simulink model "octave1"  (R2015a)
settings: Solver=ode45  StartTime=0.0  StopTime=10.0  RelTol=1e-3
InitFcn:
  | %% DSPBuilder Start
  | alt_dspbuilder_update_model(bdroot)
  | %% DSPBuilder End
libraries: allblocks_alteradspbuilder2 x1175
(part 2 of 16)

== system octave1/GradOrien/sub_GradOrian ==
  L_y_add_1 : Inport
  L_x_add_1 : Inport  Port=2
  L_x_sub_1 : Inport  Port=3
  L_y_sub_1 : Inport  Port=4
  AltBus : allblocks_alteradspbuilder2/AltBus  BusType=Unsigned Integer  bwl=9  bwr=0  saturate=off  floatingPointInput=on  floatingPointOutput=on  logOutputs=off  logFile=C:\Users\ASUS\Desktop\sift_fpga_final\Octave_1\tb_octave1\octave1_GradOrien_sub%5FGradOrian_AltBus.fixedpointlog
  Bus Builder : allblocks_alteradspbuilder2/Bus Builder  BusType=Unsigned Integer  bwl=3  bwr=1  pipeline_display=0
  Comparator3 : allblocks_alteradspbuilder2/Comparator  direction=a > b  pipeline_display=0  allowFloatingPointOverride=on  logOutputs=off  logFile=C:\Users\ASUS\Desktop\sift_fpga_final\Octave_1\tb_octave1\octave1_GradOrien_sub%5FGradOrian_Comparator3.fixedpointlog
  Comparator4 : allblocks_alteradspbuilder2/Comparator  direction=a > b  pipeline_display=0  allowFloatingPointOverride=on  logOutputs=off  logFile=C:\Users\ASUS\Desktop\sift_fpga_final\Octave_1\tb_octave1\octave1_GradOrien_sub%5FGradOrian_Comparator4.fixedpointlog
  Comparator5 : allblocks_alteradspbuilder2/Comparator  direction=a > b  pipeline_display=0  allowFloatingPointOverride=on  logOutputs=off  logFile=C:\Users\ASUS\Desktop\sift_fpga_final\Octave_1\tb_octave1\octave1_GradOrien_sub%5FGradOrian_Comparator5.fixedpointlog
  Constant : allblocks_alteradspbuilder2/Constant  mask_cst=5  BusType=Unsigned Integer  bwl=8  bwr=0  roundMode=Truncate  satMode=Wrap  SpecifyClock=off  allowFloatingPointOverride=on  logOutputs=off  logFile=C:\Users\ASUS\Desktop\sift_fpga_final\Octave_1\tb_octave1\octave1_GradOrien_sub%5FGradOrian_Constant.fixedpointlog
  Constant1 : allblocks_alteradspbuilder2/Constant  mask_cst=4  BusType=Unsigned Integer  bwl=8  bwr=0  roundMode=Truncate  satMode=Wrap  SpecifyClock=off  allowFloatingPointOverride=on  logOutputs=off  logFile=C:\Users\ASUS\Desktop\sift_fpga_final\Octave_1\tb_octave1\octave1_GradOrien_sub%5FGradOrian_Constant1.fixedpointlog
  Constant2 : allblocks_alteradspbuilder2/Constant  mask_cst=7  BusType=Unsigned Integer  bwl=8  bwr=0  roundMode=Truncate  satMode=Wrap  SpecifyClock=off  allowFloatingPointOverride=on  logOutputs=off  logFile=C:\Users\ASUS\Desktop\sift_fpga_final\Octave_1\tb_octave1\octave1_GradOrien_sub%5FGradOrian_Constant2.fixedpointlog
  Constant3 : allblocks_alteradspbuilder2/Constant  mask_cst=1  BusType=Unsigned Integer  bwl=8  bwr=0  roundMode=Truncate  satMode=Wrap  SpecifyClock=off  allowFloatingPointOverride=on  logOutputs=off  logFile=C:\Users\ASUS\Desktop\sift_fpga_final\Octave_1\tb_octave1\octave1_GradOrien_sub%5FGradOrian_Constant3.fixedpointlog
  Constant4 : allblocks_alteradspbuilder2/Constant  mask_cst=6  BusType=Unsigned Integer  bwl=8  bwr=0  roundMode=Truncate  satMode=Wrap  SpecifyClock=off  allowFloatingPointOverride=on  logOutputs=off  logFile=C:\Users\ASUS\Desktop\sift_fpga_final\Octave_1\tb_octave1\octave1_GradOrien_sub%5FGradOrian_Constant4.fixedpointlog
  Constant5 : allblocks_alteradspbuilder2/Constant  mask_cst=3  BusType=Unsigned Integer  bwl=8  bwr=0  roundMode=Truncate  satMode=Wrap  SpecifyClock=off  allowFloatingPointOverride=on  logOutputs=off  logFile=C:\Users\ASUS\Desktop\sift_fpga_final\Octave_1\tb_octave1\octave1_GradOrien_sub%5FGradOrian_Constant5.fixedpointlog
  Constant6 : allblocks_alteradspbuilder2/Constant  mask_cst=8  BusType=Unsigned Integer  bwl=8  bwr=0  roundMode=Truncate  satMode=Wrap  SpecifyClock=off  allowFloatingPointOverride=on  logOutputs=off  logFile=C:\Users\ASUS\Desktop\sift_fpga_final\Octave_1\tb_octave1\octave1_GradOrien_sub%5FGradOrian_Constant6.fixedpointlog
  Constant7 : allblocks_alteradspbuilder2/Constant  mask_cst=2  BusType=Unsigned Integer  bwl=8  bwr=0  roundMode=Truncate  satMode=Wrap  SpecifyClock=off  allowFloatingPointOverride=on  logOutputs=off  logFile=C:\Users\ASUS\Desktop\sift_fpga_final\Octave_1\tb_octave1\octave1_GradOrien_sub%5FGradOrian_Constant7.fixedpointlog
  Delay : allblocks_alteradspbuilder2/Delay  pipeline=1  pipeline_display=1  ClockPhase=1  use_ena=on  use_sclr=off  allowFloatingPointOverride=on  logOutputs=off  logFile=C:\Users\ASUS\Desktop\sift_fpga_final\Octave_1\tb_octave1\octave1_GradOrien_sub%5FGradOrian_Delay.fixedpointlog  use_init=off  reset_value=1
  Delay1 : allblocks_alteradspbuilder2/Delay  pipeline=1  pipeline_display=1  ClockPhase=1  use_ena=on  use_sclr=off  allowFloatingPointOverride=on  logOutputs=off  logFile=C:\Users\ASUS\Desktop\sift_fpga_final\Octave_1\tb_octave1\octave1_GradOrien_sub%5FGradOrian_Delay1.fixedpointlog  use_init=off  reset_value=1
  Delay2 : allblocks_alteradspbuilder2/Delay  pipeline=1  pipeline_display=1  ClockPhase=1  use_ena=on  use_sclr=off  allowFloatingPointOverride=on  logOutputs=off  logFile=C:\Users\ASUS\Desktop\sift_fpga_final\Octave_1\tb_octave1\octave1_GradOrien_sub%5FGradOrian_Delay2.fixedpointlog  use_init=off  reset_value=1
  Multiplexer2 : allblocks_alteradspbuilder2/Multiplexer  numInputs=8  pipeline=0  oneHot=off  pipeline_display=0  use_ena=off  use_aclr=off  allowFloatingPointOverride=on  logOutputs=off  logFile=C:\Users\ASUS\Desktop\sift_fpga_final\Octave_1\tb_octave1\octave1_GradOrien_sub%5FGradOrian_Multiplexer2.fixedpointlog
  Multiplexer3 : allblocks_alteradspbuilder2/Multiplexer  numInputs=2  pipeline=0  oneHot=off  pipeline_display=0  use_ena=off  use_aclr=off  allowFloatingPointOverride=on  logOutputs=off  logFile=C:\Users\ASUS\Desktop\sift_fpga_final\Octave_1\tb_octave1\octave1_GradOrien_sub%5FGradOrian_Multiplexer3.fixedpointlog
  Multiplexer4 : allblocks_alteradspbuilder2/Multiplexer  numInputs=2  pipeline=0  oneHot=off  pipeline_display=0  use_ena=off  use_aclr=off  allowFloatingPointOverride=on  logOutputs=off  logFile=C:\Users\ASUS\Desktop\sift_fpga_final\Octave_1\tb_octave1\octave1_GradOrien_sub%5FGradOrian_Multiplexer4.fixedpointlog
  Parallel Adder Subtractor : allblocks_alteradspbuilder2/Parallel Adder Subtractor  number_of_inputs=2  direction=+-  use_pipeline=on  pipeline_display=1  phase_selection=1  use_ena=on  use_aclr=off  allowFloatingPointOverride=on  logOutputs=off  logFile=C:\Users\ASUS\Desktop\sift_fpga_final\Octave_1\tb_octave1\octave1_GradOrien_sub%5FGradOrian_Parallel+Adder+Subtractor.fixedpointlog
  Parallel Adder Subtractor1 : allblocks_alteradspbuilder2/Parallel Adder Subtractor  number_of_inputs=2  direction=+-  use_pipeline=on  pipeline_display=1  phase_selection=1  use_ena=on  use_aclr=off  allowFloatingPointOverride=on  logOutputs=off  logFile=C:\Users\ASUS\Desktop\sift_fpga_final\Octave_1\tb_octave1\octave1_GradOrien_sub%5FGradOrian_Parallel+Adder+Subtractor1.fixedpointlog
  Parallel Adder Subtractor2 : allblocks_alteradspbuilder2/Parallel Adder Subtractor  number_of_inputs=2  direction=-+  use_pipeline=on  pipeline_display=1  phase_selection=1  use_ena=on  use_aclr=off  allowFloatingPointOverride=on  logOutputs=off  logFile=C:\Users\ASUS\Desktop\sift_fpga_final\Octave_1\tb_octave1\octave1_GradOrien_sub%5FGradOrian_Parallel+Adder+Subtractor2.fixedpointlog
  Parallel Adder Subtractor3 : allblocks_alteradspbuilder2/Parallel Adder Subtractor  number_of_inputs=2  direction=-+  use_pipeline=on  pipeline_display=1  phase_selection=1  use_ena=on  use_aclr=off  allowFloatingPointOverride=on  logOutputs=off  logFile=C:\Users\ASUS\Desktop\sift_fpga_final\Octave_1\tb_octave1\octave1_GradOrien_sub%5FGradOrian_Parallel+Adder+Subtractor3.fixedpointlog
  Parallel Adder Subtractor5 : allblocks_alteradspbuilder2/Parallel Adder Subtractor  number_of_inputs=2  direction=++  use_pipeline=on  pipeline_display=1  phase_selection=1  use_ena=on  use_aclr=off  allowFloatingPointOverride=on  logOutputs=off  logFile=C:\Users\ASUS\Desktop\sift_fpga_final\Octave_1\tb_octave1\octave1_GradOrien_sub%5FGradOrian_Parallel+Adder+Subtractor5.fixedpointlog
  orien : Outport
  m_xy : Outport  Port=2
  wires:
  Multiplexer2/1 -> Delay2/1
  Bus Builder/1 -> Multiplexer2/1
  Delay2/1 -> orien/1
  Constant6/1 -> Multiplexer2/8
  Constant4/1 -> Multiplexer2/6
  Constant5/1 -> Multiplexer2/7
  Comparator3/1 -> Delay/1
  Constant7/1 -> Multiplexer2/9
  [L_y_sub_1] -> Comparator4/2
  [L_x_sub_1] -> Comparator3/2
  [L_y_add_1] -> Comparator4/1
  [L_x_add_1] -> Comparator3/1
  [Ly_1] -> Multiplexer4/2
  Delay1/1 -> Bus Builder/2, Multiplexer4/1
  [Lx] -> Multiplexer3/3
  Delay/1 -> Bus Builder/1, Multiplexer3/1
  [Lx_1] -> Multiplexer3/2
  [Ly] -> Multiplexer4/3
  Constant/1 -> Multiplexer2/2
  [clken] -> Delay1/2
  Comparator5/1 -> Bus Builder/3
  [clken] -> Delay/2
  Comparator4/1 -> Delay1/1
  Multiplexer4/1 -> Comparator5/2, Parallel Adder Subtractor5/2
  Multiplexer3/1 -> Comparator5/1, Parallel Adder Subtractor5/1
  [clken] -> Parallel Adder Subtractor5/3
  Parallel Adder Subtractor5/1 -> AltBus/1
  [clken] -> Delay2/2
  Constant1/1 -> Multiplexer2/3
  Parallel Adder Subtractor2/1 -> [Lx_1]
  [clken] -> Parallel Adder Subtractor2/3
  [L_y_add_1] -> Parallel Adder Subtractor3/1
  Parallel Adder Subtractor3/1 -> [Ly_1]
  [L_y_sub_1] -> Parallel Adder Subtractor3/2
  [L_x_sub_1] -> Parallel Adder Subtractor2/2
  [clken] -> Parallel Adder Subtractor3/3
  [L_x_add_1] -> Parallel Adder Subtractor2/1
  [L_x_sub_1] -> Parallel Adder Subtractor/2
  [L_y_sub_1] -> Parallel Adder Subtractor1/2
  [L_y_add_1] -> Parallel Adder Subtractor1/1
  [clken] -> Parallel Adder Subtractor/3
  Parallel Adder Subtractor/1 -> [Lx]
  Parallel Adder Subtractor1/1 -> [Ly]
  [clken] -> Parallel Adder Subtractor1/3
  [L_x_add_1] -> Parallel Adder Subtractor/1
  Constant2/1 -> Multiplexer2/4
  Constant3/1 -> Multiplexer2/5
  L_x_add_1/1 -> [L_x_add_1]
  L_x_sub_1/1 -> [L_x_sub_1]
  L_y_add_1/1 -> [L_y_add_1]
  L_y_sub_1/1 -> [L_y_sub_1]
  AltBus/1 -> m_xy/1

== system octave1/calculate_key_point/find_KeyPoint ==
  dataIn_10 : Inport
  dataIn_11 : Inport  Port=2
  dataIn_12 : Inport  Port=3
  dataIn_13 : Inport  Port=4
  dataIn_14 : Inport  Port=5
  dataIn_15 : Inport  Port=6
  dataIn_16 : Inport  Port=7
  dataIn_17 : Inport  Port=8
  dataIn_18 : Inport  Port=9
  dataIn_20 : Inport  Port=10
  dataIn_21 : Inport  Port=11
  dataIn_22 : Inport  Port=12
  dataIn_23 : Inport  Port=13
  dataIn_24 : Inport  Port=14
  dataIn_25 : Inport  Port=15
  dataIn_26 : Inport  Port=16
  dataIn_27 : Inport  Port=17
  dataIn_28 : Inport  Port=18
  dataIn_30 : Inport  Port=19
  dataIn_31 : Inport  Port=20
  dataIn_32 : Inport  Port=21
  dataIn_33 : Inport  Port=22
  dataIn_34 : Inport  Port=23
  dataIn_35 : Inport  Port=24
  dataIn_36 : Inport  Port=25
  dataIn_37 : Inport  Port=26
  dataIn_38 : Inport  Port=27
  Logical Bit Operator : allblocks_alteradspbuilder2/Logical Bit Operator  LogicalOperator=OR  user_inputs=2  pipeline_display=0
  find_Keymax : Subsystem
  find_min : Subsystem
  is_KeyPoint : Outport
  wires:
  [dataIn_32] -> find_Keymax/21(dataIn_32)
  [dataIn_33] -> find_Keymax/22(dataIn_33)
  [dataIn_36] -> find_Keymax/25(dataIn_36)
  [dataIn_37] -> find_Keymax/26(dataIn_37)
  [dataIn_34] -> find_Keymax/23(dataIn_34)
  [dataIn_35] -> find_Keymax/24(dataIn_35)
  [dataIn_30] -> find_Keymax/19(dataIn_30)
  [dataIn_31] -> find_Keymax/20(dataIn_31)
  [is_KeyPoint_Max] -> Logical Bit Operator/2
  [is_KeyPoint_Min] -> Logical Bit Operator/1
  find_Keymax/1(is_KeyPoint) -> [is_KeyPoint_Max]
  [dataIn_28] -> find_Keymax/18(dataIn_28)
  [dataIn_26] -> find_Keymax/16(dataIn_26)
  [dataIn_22] -> find_Keymax/12(dataIn_22)
  [dataIn_27] -> find_Keymax/17(dataIn_27)
  [dataIn_20] -> find_Keymax/10(dataIn_20)
  [dataIn_23] -> find_Keymax/13(dataIn_23)
  [dataIn_24] -> find_Keymax/14(dataIn_24)
  [dataIn_21] -> find_Keymax/11(dataIn_21)
  [dataIn_25] -> find_Keymax/15(dataIn_25)
  [dataIn_10] -> find_Keymax/1(dataIn_10)
  [dataIn_11] -> find_Keymax/2(dataIn_11)
  [dataIn_12] -> find_Keymax/3(dataIn_12)
  dataIn_23/1 -> [dataIn_23]
  dataIn_17/1 -> [dataIn_17]
  dataIn_22/1 -> [dataIn_22]
  dataIn_14/1 -> [dataIn_14]
  dataIn_16/1 -> [dataIn_16]
  dataIn_28/1 -> [dataIn_28]
  dataIn_20/1 -> [dataIn_20]
  dataIn_21/1 -> [dataIn_21]
  dataIn_26/1 -> [dataIn_26]
  dataIn_10/1 -> [dataIn_10]
  dataIn_30/1 -> [dataIn_30]
  dataIn_27/1 -> [dataIn_27]
  dataIn_25/1 -> [dataIn_25]
  dataIn_15/1 -> [dataIn_15]
  dataIn_18/1 -> [dataIn_18]
  dataIn_24/1 -> [dataIn_24]
  dataIn_32/1 -> [dataIn_32]
  dataIn_13/1 -> [dataIn_13]
  dataIn_31/1 -> [dataIn_31]
  [dataIn_14] -> find_Keymax/5(dataIn_14)
  dataIn_34/1 -> [dataIn_34]
  dataIn_11/1 -> [dataIn_11]
  [dataIn_17] -> find_Keymax/8(dataIn_17)
  dataIn_35/1 -> [dataIn_35]
  dataIn_33/1 -> [dataIn_33]
  dataIn_38/1 -> [dataIn_38]
  [dataIn_13] -> find_Keymax/4(dataIn_13)
  [dataIn_16] -> find_Keymax/7(dataIn_16)
  [dataIn_15] -> find_Keymax/6(dataIn_15)
  dataIn_12/1 -> [dataIn_12]
  [dataIn_18] -> find_Keymax/9(dataIn_18)
  dataIn_36/1 -> [dataIn_36]
  dataIn_37/1 -> [dataIn_37]
  [dataIn_38] -> find_Keymax/27(dataIn_38)
  find_min/1(is_KeyPoint) -> [is_KeyPoint_Min]
  [dataIn_11] -> find_min/2(dataIn_11)
  [dataIn_12] -> find_min/3(dataIn_12)
  [dataIn_13] -> find_min/4(dataIn_13)
  [dataIn_15] -> find_min/6(dataIn_15)
  [dataIn_16] -> find_min/7(dataIn_16)
  [dataIn_17] -> find_min/8(dataIn_17)
  [dataIn_18] -> find_min/9(dataIn_18)
  [dataIn_31] -> find_min/20(dataIn_31)
  [dataIn_14] -> find_min/5(dataIn_14)
  [is_KeyPoint] -> is_KeyPoint/1
  [dataIn_33] -> find_min/22(dataIn_33)
  [dataIn_32] -> find_min/21(dataIn_32)
  [dataIn_34] -> find_min/23(dataIn_34)
  [dataIn_35] -> find_min/24(dataIn_35)
  [dataIn_36] -> find_min/25(dataIn_36)
  [dataIn_21] -> find_min/11(dataIn_21)
  [dataIn_22] -> find_min/12(dataIn_22)
  [dataIn_23] -> find_min/13(dataIn_23)
  [dataIn_25] -> find_min/15(dataIn_25)
  [dataIn_24] -> find_min/14(dataIn_24)
  [dataIn_38] -> find_min/27(dataIn_38)
  [dataIn_20] -> find_min/10(dataIn_20)
  [dataIn_26] -> find_min/16(dataIn_26)
  [dataIn_30] -> find_min/19(dataIn_30)
  [dataIn_27] -> find_min/17(dataIn_27)
  [dataIn_37] -> find_min/26(dataIn_37)
  [dataIn_28] -> find_min/18(dataIn_28)
  [dataIn_10] -> find_min/1(dataIn_10)
  Logical Bit Operator/1 -> [is_KeyPoint]

== system octave1/calculate_key_point/line_buff_3x3 ==
  dataIn : Inport
  clken : Inport  Port=2
  Delay : allblocks_alteradspbuilder2/Delay  pipeline=1  pipeline_display=1  ClockPhase=1  use_ena=on  use_sclr=off  allowFloatingPointOverride=on  logOutputs=off  logFile=C:\Users\ASUS\Desktop\sift_fpga_final\Octave_1\find_key_point\tb_calculate_key_points\calculate%5Fkey%5Fpoints_calculate%5Fkey%5Fpoint_line%5Fbuff%5F3x3_Delay.fixedpointlog  use_init=off  reset_value=1
  Delay1 : allblocks_alteradspbuilder2/Delay  pipeline=1  pipeline_display=1  ClockPhase=1  use_ena=on  use_sclr=off  allowFloatingPointOverride=on  logOutputs=off  logFile=C:\Users\ASUS\Desktop\sift_fpga_final\Octave_1\find_key_point\tb_calculate_key_points\calculate%5Fkey%5Fpoints_calculate%5Fkey%5Fpoint_line%5Fbuff%5F3x3_Delay1.fixedpointlog  use_init=off  reset_value=1
  Delay10 : allblocks_alteradspbuilder2/Delay  pipeline=1  pipeline_display=1  ClockPhase=1  use_ena=on  use_sclr=off  allowFloatingPointOverride=on  logOutputs=off  logFile=C:\Users\ASUS\Desktop\sift_fpga_final\Octave_1\find_key_point\tb_calculate_key_points\calculate%5Fkey%5Fpoints_calculate%5Fkey%5Fpoint_line%5Fbuff%5F3x3_Delay10.fixedpointlog  use_init=off  reset_value=1
  Delay2 : allblocks_alteradspbuilder2/Delay  pipeline=1  pipeline_display=1  ClockPhase=1  use_ena=on  use_sclr=off  allowFloatingPointOverride=on  logOutputs=off  logFile=C:\Users\ASUS\Desktop\sift_fpga_final\Octave_1\find_key_point\tb_calculate_key_points\calculate%5Fkey%5Fpoints_calculate%5Fkey%5Fpoint_line%5Fbuff%5F3x3_Delay2.fixedpointlog  use_init=off  reset_value=1
  Delay5 : allblocks_alteradspbuilder2/Delay  pipeline=1  pipeline_display=1  ClockPhase=1  use_ena=on  use_sclr=off  allowFloatingPointOverride=on  logOutputs=off  logFile=C:\Users\ASUS\Desktop\sift_fpga_final\Octave_1\find_key_point\tb_calculate_key_points\calculate%5Fkey%5Fpoints_calculate%5Fkey%5Fpoint_line%5Fbuff%5F3x3_Delay5.fixedpointlog  use_init=off  reset_value=1
  Delay6 : allblocks_alteradspbuilder2/Delay  pipeline=1  pipeline_display=1  ClockPhase=1  use_ena=on  use_sclr=off  allowFloatingPointOverride=on  logOutputs=off  logFile=C:\Users\ASUS\Desktop\sift_fpga_final\Octave_1\find_key_point\tb_calculate_key_points\calculate%5Fkey%5Fpoints_calculate%5Fkey%5Fpoint_line%5Fbuff%5F3x3_Delay6.fixedpointlog  use_init=off  reset_value=1
  Delay9 : allblocks_alteradspbuilder2/Delay  pipeline=1  pipeline_display=1  ClockPhase=1  use_ena=on  use_sclr=off  allowFloatingPointOverride=on  logOutputs=off  logFile=C:\Users\ASUS\Desktop\sift_fpga_final\Octave_1\find_key_point\tb_calculate_key_points\calculate%5Fkey%5Fpoints_calculate%5Fkey%5Fpoint_line%5Fbuff%5F3x3_Delay9.fixedpointlog  use_init=off  reset_value=1
  Memory Delay : allblocks_alteradspbuilder2/Memory Delay  BusType=Unsigned Integer  bwl=8  bwr=0  pipeline=638  pipeline_display=638  ram_type=AUTO  use_ena=on  use_sclr=off  allowFloatingPointOverride=on  logOutputs=off  logFile=C:\Users\ASUS\Desktop\sift_fpga_final\Octave_1\find_key_point\tb_calculate_key_points\calculate%5Fkey%5Fpoints_calculate%5Fkey%5Fpoint_line%5Fbuff%5F3x3_Memory+Delay.fixedpointlog
  Memory Delay1 : allblocks_alteradspbuilder2/Memory Delay  BusType=Unsigned Integer  bwl=8  bwr=0  pipeline=638  pipeline_display=638  ram_type=AUTO  use_ena=on  use_sclr=off  allowFloatingPointOverride=on  logOutputs=off  logFile=C:\Users\ASUS\Desktop\sift_fpga_final\Octave_1\find_key_point\tb_calculate_key_points\calculate%5Fkey%5Fpoints_calculate%5Fkey%5Fpoint_line%5Fbuff%5F3x3_Memory+Delay1.fixedpointlog
  Out00 : Outport
  Out01 : Outport  Port=2
  Out02 : Outport  Port=3
  Out10 : Outport  Port=4
  Out11 : Outport  Port=5
  Out12 : Outport  Port=6
  Out20 : Outport  Port=7
  Out21 : Outport  Port=8
  Out22 : Outport  Port=9
  wires:
  Delay1/1 -> [data_01], Delay2/1
  Delay/1 -> [data_00], Delay1/1
  Delay9/1 -> [data_21], Delay10/1
  [clken] -> Delay10/2
  [clken] -> Memory Delay1/2
  Delay6/1 -> Memory Delay1/1, [data_12]
  Memory Delay1/1 -> [data_20], Delay9/1
  [clken] -> Delay9/2
  [data_02] -> Out02/1
  [clken] -> Delay1/2
  [clken] -> Delay/2
  [data_in] -> Delay/1
  [clken] -> Delay2/2
  Delay2/1 -> Memory Delay/1, [data_02]
  [data_22] -> Out22/1
  Delay10/1 -> [data_22]
  clken/1 -> [clken]
  [data_21] -> Out21/1
  [data_20] -> Out20/1
  [data_10] -> Out10/1
  Memory Delay/1 -> [data_10], Delay5/1
  [clken] -> Memory Delay/2
  [clken] -> Delay6/2
  Delay5/1 -> [data_11], Delay6/1
  [data_12] -> Out12/1
  [data_00] -> Out00/1
  [data_01] -> Out01/1
  [clken] -> Delay5/2
  [data_11] -> Out11/1
  dataIn/1 -> [data_in]

== system octave1/calculate_key_point/line_buff_3x3(1) ==
  dataIn : Inport
  clken : Inport  Port=2
  Delay : allblocks_alteradspbuilder2/Delay  pipeline=1  pipeline_display=1  ClockPhase=1  use_ena=on  use_sclr=off  allowFloatingPointOverride=on  logOutputs=off  logFile=C:\Users\ASUS\Desktop\sift_fpga_final\Octave_1\find_key_point\tb_calculate_key_points\calculate%5Fkey%5Fpoints_calculate%5Fkey%5Fpoint_line%5Fbuff%5F3x3%281%29_Delay.fixedpointlog  use_init=off  reset_value=1
  Delay1 : allblocks_alteradspbuilder2/Delay  pipeline=1  pipeline_display=1  ClockPhase=1  use_ena=on  use_sclr=off  allowFloatingPointOverride=on  logOutputs=off  logFile=C:\Users\ASUS\Desktop\sift_fpga_final\Octave_1\find_key_point\tb_calculate_key_points\calculate%5Fkey%5Fpoints_calculate%5Fkey%5Fpoint_line%5Fbuff%5F3x3%281%29_Delay1.fixedpointlog  use_init=off  reset_value=1
  Delay10 : allblocks_alteradspbuilder2/Delay  pipeline=1  pipeline_display=1  ClockPhase=1  use_ena=on  use_sclr=off  allowFloatingPointOverride=on  logOutputs=off  logFile=C:\Users\ASUS\Desktop\sift_fpga_final\Octave_1\find_key_point\tb_calculate_key_points\calculate%5Fkey%5Fpoints_calculate%5Fkey%5Fpoint_line%5Fbuff%5F3x3%281%29_Delay10.fixedpointlog  use_init=off  reset_value=1
  Delay2 : allblocks_alteradspbuilder2/Delay  pipeline=1  pipeline_display=1  ClockPhase=1  use_ena=on  use_sclr=off  allowFloatingPointOverride=on  logOutputs=off  logFile=C:\Users\ASUS\Desktop\sift_fpga_final\Octave_1\find_key_point\tb_calculate_key_points\calculate%5Fkey%5Fpoints_calculate%5Fkey%5Fpoint_line%5Fbuff%5F3x3%281%29_Delay2.fixedpointlog  use_init=off  reset_value=1
  Delay5 : allblocks_alteradspbuilder2/Delay  pipeline=1  pipeline_display=1  ClockPhase=1  use_ena=on  use_sclr=off  allowFloatingPointOverride=on  logOutputs=off  logFile=C:\Users\ASUS\Desktop\sift_fpga_final\Octave_1\find_key_point\tb_calculate_key_points\calculate%5Fkey%5Fpoints_calculate%5Fkey%5Fpoint_line%5Fbuff%5F3x3%281%29_Delay5.fixedpointlog  use_init=off  reset_value=1
  Delay6 : allblocks_alteradspbuilder2/Delay  pipeline=1  pipeline_display=1  ClockPhase=1  use_ena=on  use_sclr=off  allowFloatingPointOverride=on  logOutputs=off  logFile=C:\Users\ASUS\Desktop\sift_fpga_final\Octave_1\find_key_point\tb_calculate_key_points\calculate%5Fkey%5Fpoints_calculate%5Fkey%5Fpoint_line%5Fbuff%5F3x3%281%29_Delay6.fixedpointlog  use_init=off  reset_value=1
  Delay9 : allblocks_alteradspbuilder2/Delay  pipeline=1  pipeline_display=1  ClockPhase=1  use_ena=on  use_sclr=off  allowFloatingPointOverride=on  logOutputs=off  logFile=C:\Users\ASUS\Desktop\sift_fpga_final\Octave_1\find_key_point\tb_calculate_key_points\calculate%5Fkey%5Fpoints_calculate%5Fkey%5Fpoint_line%5Fbuff%5F3x3%281%29_Delay9.fixedpointlog  use_init=off  reset_value=1
  Memory Delay : allblocks_alteradspbuilder2/Memory Delay  BusType=Unsigned Integer  bwl=8  bwr=0  pipeline=638  pipeline_display=638  ram_type=AUTO  use_ena=on  use_sclr=off  allowFloatingPointOverride=on  logOutputs=off  logFile=C:\Users\ASUS\Desktop\sift_fpga_final\Octave_1\find_key_point\tb_calculate_key_points\calculate%5Fkey%5Fpoints_calculate%5Fkey%5Fpoint_line%5Fbuff%5F3x3%281%29_Memory+Delay.fixedpointlog
  Memory Delay1 : allblocks_alteradspbuilder2/Memory Delay  BusType=Unsigned Integer  bwl=8  bwr=0  pipeline=638  pipeline_display=638  ram_type=AUTO  use_ena=on  use_sclr=off  allowFloatingPointOverride=on  logOutputs=off  logFile=C:\Users\ASUS\Desktop\sift_fpga_final\Octave_1\find_key_point\tb_calculate_key_points\calculate%5Fkey%5Fpoints_calculate%5Fkey%5Fpoint_line%5Fbuff%5F3x3%281%29_Memory+Delay1.fixedpointlog
  Out00 : Outport
  Out01 : Outport  Port=2
  Out02 : Outport  Port=3
  Out10 : Outport  Port=4
  Out11 : Outport  Port=5
  Out12 : Outport  Port=6
  Out20 : Outport  Port=7
  Out21 : Outport  Port=8
  Out22 : Outport  Port=9
  wires:
  Delay1/1 -> [data_01], Delay2/1
  Delay/1 -> [data_00], Delay1/1
  Delay9/1 -> [data_21], Delay10/1
  [clken] -> Delay10/2
  [clken] -> Memory Delay1/2
  Delay6/1 -> Memory Delay1/1, [data_12]
  Memory Delay1/1 -> [data_20], Delay9/1
  [clken] -> Delay9/2
  [data_02] -> Out02/1
  [clken] -> Delay1/2
  [clken] -> Delay/2
  [data_in] -> Delay/1
  [clken] -> Delay2/2
  Delay2/1 -> Memory Delay/1, [data_02]
  [data_22] -> Out22/1
  Delay10/1 -> [data_22]
  clken/1 -> [clken]
  [data_21] -> Out21/1
  [data_20] -> Out20/1
  [data_10] -> Out10/1
  Memory Delay/1 -> [data_10], Delay5/1
  [clken] -> Memory Delay/2
  [clken] -> Delay6/2
  Delay5/1 -> [data_11], Delay6/1
  [data_12] -> Out12/1
  [data_00] -> Out00/1
  [data_01] -> Out01/1
  [clken] -> Delay5/2
  [data_11] -> Out11/1
  dataIn/1 -> [data_in]

== system octave1/calculate_key_point/line_buff_3x3(2) ==
  dataIn : Inport
  clken : Inport  Port=2
  Delay : allblocks_alteradspbuilder2/Delay  pipeline=1  pipeline_display=1  ClockPhase=1  use_ena=on  use_sclr=off  allowFloatingPointOverride=on  logOutputs=off  logFile=C:\Users\ASUS\Desktop\sift_fpga_final\Octave_1\find_key_point\tb_calculate_key_points\calculate%5Fkey%5Fpoints_calculate%5Fkey%5Fpoint_line%5Fbuff%5F3x3%282%29_Delay.fixedpointlog  use_init=off  reset_value=1
  Delay1 : allblocks_alteradspbuilder2/Delay  pipeline=1  pipeline_display=1  ClockPhase=1  use_ena=on  use_sclr=off  allowFloatingPointOverride=on  logOutputs=off  logFile=C:\Users\ASUS\Desktop\sift_fpga_final\Octave_1\find_key_point\tb_calculate_key_points\calculate%5Fkey%5Fpoints_calculate%5Fkey%5Fpoint_line%5Fbuff%5F3x3%282%29_Delay1.fixedpointlog  use_init=off  reset_value=1
  Delay10 : allblocks_alteradspbuilder2/Delay  pipeline=1  pipeline_display=1  ClockPhase=1  use_ena=on  use_sclr=off  allowFloatingPointOverride=on  logOutputs=off  logFile=C:\Users\ASUS\Desktop\sift_fpga_final\Octave_1\find_key_point\tb_calculate_key_points\calculate%5Fkey%5Fpoints_calculate%5Fkey%5Fpoint_line%5Fbuff%5F3x3%282%29_Delay10.fixedpointlog  use_init=off  reset_value=1
  Delay2 : allblocks_alteradspbuilder2/Delay  pipeline=1  pipeline_display=1  ClockPhase=1  use_ena=on  use_sclr=off  allowFloatingPointOverride=on  logOutputs=off  logFile=C:\Users\ASUS\Desktop\sift_fpga_final\Octave_1\find_key_point\tb_calculate_key_points\calculate%5Fkey%5Fpoints_calculate%5Fkey%5Fpoint_line%5Fbuff%5F3x3%282%29_Delay2.fixedpointlog  use_init=off  reset_value=1
  Delay5 : allblocks_alteradspbuilder2/Delay  pipeline=1  pipeline_display=1  ClockPhase=1  use_ena=on  use_sclr=off  allowFloatingPointOverride=on  logOutputs=off  logFile=C:\Users\ASUS\Desktop\sift_fpga_final\Octave_1\find_key_point\tb_calculate_key_points\calculate%5Fkey%5Fpoints_calculate%5Fkey%5Fpoint_line%5Fbuff%5F3x3%282%29_Delay5.fixedpointlog  use_init=off  reset_value=1
  Delay6 : allblocks_alteradspbuilder2/Delay  pipeline=1  pipeline_display=1  ClockPhase=1  use_ena=on  use_sclr=off  allowFloatingPointOverride=on  logOutputs=off  logFile=C:\Users\ASUS\Desktop\sift_fpga_final\Octave_1\find_key_point\tb_calculate_key_points\calculate%5Fkey%5Fpoints_calculate%5Fkey%5Fpoint_line%5Fbuff%5F3x3%282%29_Delay6.fixedpointlog  use_init=off  reset_value=1
  Delay9 : allblocks_alteradspbuilder2/Delay  pipeline=1  pipeline_display=1  ClockPhase=1  use_ena=on  use_sclr=off  allowFloatingPointOverride=on  logOutputs=off  logFile=C:\Users\ASUS\Desktop\sift_fpga_final\Octave_1\find_key_point\tb_calculate_key_points\calculate%5Fkey%5Fpoints_calculate%5Fkey%5Fpoint_line%5Fbuff%5F3x3%282%29_Delay9.fixedpointlog  use_init=off  reset_value=1
  Memory Delay : allblocks_alteradspbuilder2/Memory Delay  BusType=Unsigned Integer  bwl=8  bwr=0  pipeline=638  pipeline_display=638  ram_type=AUTO  use_ena=on  use_sclr=off  allowFloatingPointOverride=on  logOutputs=off  logFile=C:\Users\ASUS\Desktop\sift_fpga_final\Octave_1\find_key_point\tb_calculate_key_points\calculate%5Fkey%5Fpoints_calculate%5Fkey%5Fpoint_line%5Fbuff%5F3x3%282%29_Memory+Delay.fixedpointlog
  Memory Delay1 : allblocks_alteradspbuilder2/Memory Delay  BusType=Unsigned Integer  bwl=8  bwr=0  pipeline=638  pipeline_display=638  ram_type=AUTO  use_ena=on  use_sclr=off  allowFloatingPointOverride=on  logOutputs=off  logFile=C:\Users\ASUS\Desktop\sift_fpga_final\Octave_1\find_key_point\tb_calculate_key_points\calculate%5Fkey%5Fpoints_calculate%5Fkey%5Fpoint_line%5Fbuff%5F3x3%282%29_Memory+Delay1.fixedpointlog
  Out00 : Outport
  Out01 : Outport  Port=2
  Out02 : Outport  Port=3
  Out10 : Outport  Port=4
  Out11 : Outport  Port=5
  Out12 : Outport  Port=6
  Out20 : Outport  Port=7
  Out21 : Outport  Port=8
  Out22 : Outport  Port=9
  wires:
  Delay1/1 -> [data_01], Delay2/1
  Delay/1 -> [data_00], Delay1/1
  Delay9/1 -> [data_21], Delay10/1
  [clken] -> Delay10/2
  [clken] -> Memory Delay1/2
  Delay6/1 -> Memory Delay1/1, [data_12]
  Memory Delay1/1 -> [data_20], Delay9/1
  [clken] -> Delay9/2
  [data_02] -> Out02/1
  [clken] -> Delay1/2
  [clken] -> Delay/2
  [data_in] -> Delay/1
  [clken] -> Delay2/2
  Delay2/1 -> Memory Delay/1, [data_02]
  [data_22] -> Out22/1
  Delay10/1 -> [data_22]
  clken/1 -> [clken]
  [data_21] -> Out21/1
  [data_20] -> Out20/1
  [data_10] -> Out10/1
  Memory Delay/1 -> [data_10], Delay5/1
  [clken] -> Memory Delay/2
  [clken] -> Delay6/2
  Delay5/1 -> [data_11], Delay6/1
  [data_12] -> Out12/1
  [data_00] -> Out00/1
  [data_01] -> Out01/1
  [clken] -> Delay5/2
  [data_11] -> Out11/1
  dataIn/1 -> [data_in]

== system octave1/hist_bin/Line_buffer_5x5 ==
  dataIn : Inport
  clken : Inport  Port=2
  Delay : allblocks_alteradspbuilder2/Delay  pipeline=1  pipeline_display=1  ClockPhase=1  use_ena=on  use_sclr=off  allowFloatingPointOverride=on  logOutputs=off  logFile=C:\Users\ASUS\Desktop\sift_fpga_final\Octave_1\tb_octave1\octave1_hist%5Fbin_Line%5Fbuffer%5F5x5_Delay.fixedpointlog  use_init=off  reset_value=1
  Delay1 : allblocks_alteradspbuilder2/Delay  pipeline=1  pipeline_display=1  ClockPhase=1  use_ena=on  use_sclr=off  allowFloatingPointOverride=on  logOutputs=off  logFile=C:\Users\ASUS\Desktop\sift_fpga_final\Octave_1\tb_octave1\octave1_hist%5Fbin_Line%5Fbuffer%5F5x5_Delay1.fixedpointlog  use_init=off  reset_value=1
  Delay10 : allblocks_alteradspbuilder2/Delay  pipeline=1  pipeline_display=1  ClockPhase=1  use_ena=on  use_sclr=off  allowFloatingPointOverride=on  logOutputs=off  logFile=C:\Users\ASUS\Desktop\sift_fpga_final\Octave_1\tb_octave1\octave1_hist%5Fbin_Line%5Fbuffer%5F5x5_Delay10.fixedpointlog  use_init=off  reset_value=1
  Delay11 : allblocks_alteradspbuilder2/Delay  pipeline=1  pipeline_display=1  ClockPhase=1  use_ena=on  use_sclr=off  allowFloatingPointOverride=on  logOutputs=off  logFile=C:\Users\ASUS\Desktop\sift_fpga_final\Octave_1\tb_octave1\octave1_hist%5Fbin_Line%5Fbuffer%5F5x5_Delay11.fixedpointlog  use_init=off  reset_value=1
  Delay12 : allblocks_alteradspbuilder2/Delay  pipeline=1  pipeline_display=1  ClockPhase=1  use_ena=on  use_sclr=off  allowFloatingPointOverride=on  logOutputs=off  logFile=C:\Users\ASUS\Desktop\sift_fpga_final\Octave_1\tb_octave1\octave1_hist%5Fbin_Line%5Fbuffer%5F5x5_Delay12.fixedpointlog  use_init=off  reset_value=1
  Delay13 : allblocks_alteradspbuilder2/Delay  pipeline=1  pipeline_display=1  ClockPhase=1  use_ena=on  use_sclr=off  allowFloatingPointOverride=on  logOutputs=off  logFile=C:\Users\ASUS\Desktop\sift_fpga_final\Octave_1\tb_octave1\octave1_hist%5Fbin_Line%5Fbuffer%5F5x5_Delay13.fixedpointlog  use_init=off  reset_value=1
  Delay14 : allblocks_alteradspbuilder2/Delay  pipeline=1  pipeline_display=1  ClockPhase=1  use_ena=on  use_sclr=off  allowFloatingPointOverride=on  logOutputs=off  logFile=C:\Users\ASUS\Desktop\sift_fpga_final\Octave_1\tb_octave1\octave1_hist%5Fbin_Line%5Fbuffer%5F5x5_Delay14.fixedpointlog  use_init=off  reset_value=1
  Delay15 : allblocks_alteradspbuilder2/Delay  pipeline=1  pipeline_display=1  ClockPhase=1  use_ena=on  use_sclr=off  allowFloatingPointOverride=on  logOutputs=off  logFile=C:\Users\ASUS\Desktop\sift_fpga_final\Octave_1\tb_octave1\octave1_hist%5Fbin_Line%5Fbuffer%5F5x5_Delay15.fixedpointlog  use_init=off  reset_value=1
  Delay16 : allblocks_alteradspbuilder2/Delay  pipeline=1  pipeline_display=1  ClockPhase=1  use_ena=on  use_sclr=off  allowFloatingPointOverride=on  logOutputs=off  logFile=C:\Users\ASUS\Desktop\sift_fpga_final\Octave_1\tb_octave1\octave1_hist%5Fbin_Line%5Fbuffer%5F5x5_Delay16.fixedpointlog  use_init=off  reset_value=1
  Delay17 : allblocks_alteradspbuilder2/Delay  pipeline=1  pipeline_display=1  ClockPhase=1  use_ena=on  use_sclr=off  allowFloatingPointOverride=on  logOutputs=off  logFile=C:\Users\ASUS\Desktop\sift_fpga_final\Octave_1\tb_octave1\octave1_hist%5Fbin_Line%5Fbuffer%5F5x5_Delay17.fixedpointlog  use_init=off  reset_value=1
  Delay18 : allblocks_alteradspbuilder2/Delay  pipeline=1  pipeline_display=1  ClockPhase=1  use_ena=on  use_sclr=off  allowFloatingPointOverride=on  logOutputs=off  logFile=C:\Users\ASUS\Desktop\sift_fpga_final\Octave_1\tb_octave1\octave1_hist%5Fbin_Line%5Fbuffer%5F5x5_Delay18.fixedpointlog  use_init=off  reset_value=1
  Delay19 : allblocks_alteradspbuilder2/Delay  pipeline=1  pipeline_display=1  ClockPhase=1  use_ena=on  use_sclr=off  allowFloatingPointOverride=on  logOutputs=off  logFile=C:\Users\ASUS\Desktop\sift_fpga_final\Octave_1\tb_octave1\octave1_hist%5Fbin_Line%5Fbuffer%5F5x5_Delay19.fixedpointlog  use_init=off  reset_value=1
  Delay2 : allblocks_alteradspbuilder2/Delay  pipeline=1  pipeline_display=1  ClockPhase=1  use_ena=on  use_sclr=off  allowFloatingPointOverride=on  logOutputs=off  logFile=C:\Users\ASUS\Desktop\sift_fpga_final\Octave_1\tb_octave1\octave1_hist%5Fbin_Line%5Fbuffer%5F5x5_Delay2.fixedpointlog  use_init=off  reset_value=1
  Delay20 : allblocks_alteradspbuilder2/Delay  pipeline=1  pipeline_display=1  ClockPhase=1  use_ena=on  use_sclr=off  allowFloatingPointOverride=on  logOutputs=off  logFile=C:\Users\ASUS\Desktop\sift_fpga_final\Octave_1\tb_octave1\octave1_hist%5Fbin_Line%5Fbuffer%5F5x5_Delay20.fixedpointlog  use_init=off  reset_value=1
  Delay3 : allblocks_alteradspbuilder2/Delay  pipeline=1  pipeline_display=1  ClockPhase=1  use_ena=on  use_sclr=off  allowFloatingPointOverride=on  logOutputs=off  logFile=C:\Users\ASUS\Desktop\sift_fpga_final\Octave_1\tb_octave1\octave1_hist%5Fbin_Line%5Fbuffer%5F5x5_Delay3.fixedpointlog  use_init=off  reset_value=1
  Delay4 : allblocks_alteradspbuilder2/Delay  pipeline=1  pipeline_display=1  ClockPhase=1  use_ena=on  use_sclr=off  allowFloatingPointOverride=on  logOutputs=off  logFile=C:\Users\ASUS\Desktop\sift_fpga_final\Octave_1\tb_octave1\octave1_hist%5Fbin_Line%5Fbuffer%5F5x5_Delay4.fixedpointlog  use_init=off  reset_value=1
  Delay5 : allblocks_alteradspbuilder2/Delay  pipeline=1  pipeline_display=1  ClockPhase=1  use_ena=on  use_sclr=off  allowFloatingPointOverride=on  logOutputs=off  logFile=C:\Users\ASUS\Desktop\sift_fpga_final\Octave_1\tb_octave1\octave1_hist%5Fbin_Line%5Fbuffer%5F5x5_Delay5.fixedpointlog  use_init=off  reset_value=1
  Delay6 : allblocks_alteradspbuilder2/Delay  pipeline=1  pipeline_display=1  ClockPhase=1  use_ena=on  use_sclr=off  allowFloatingPointOverride=on  logOutputs=off  logFile=C:\Users\ASUS\Desktop\sift_fpga_final\Octave_1\tb_octave1\octave1_hist%5Fbin_Line%5Fbuffer%5F5x5_Delay6.fixedpointlog  use_init=off  reset_value=1
  Delay7 : allblocks_alteradspbuilder2/Delay  pipeline=1  pipeline_display=1  ClockPhase=1  use_ena=on  use_sclr=off  allowFloatingPointOverride=on  logOutputs=off  logFile=C:\Users\ASUS\Desktop\sift_fpga_final\Octave_1\tb_octave1\octave1_hist%5Fbin_Line%5Fbuffer%5F5x5_Delay7.fixedpointlog  use_init=off  reset_value=1
  Delay8 : allblocks_alteradspbuilder2/Delay  pipeline=1  pipeline_display=1  ClockPhase=1  use_ena=on  use_sclr=off  allowFloatingPointOverride=on  logOutputs=off  logFile=C:\Users\ASUS\Desktop\sift_fpga_final\Octave_1\tb_octave1\octave1_hist%5Fbin_Line%5Fbuffer%5F5x5_Delay8.fixedpointlog  use_init=off  reset_value=1
  Delay9 : allblocks_alteradspbuilder2/Delay  pipeline=1  pipeline_display=1  ClockPhase=1  use_ena=on  use_sclr=off  allowFloatingPointOverride=on  logOutputs=off  logFile=C:\Users\ASUS\Desktop\sift_fpga_final\Octave_1\tb_octave1\octave1_hist%5Fbin_Line%5Fbuffer%5F5x5_Delay9.fixedpointlog  use_init=off  reset_value=1
  Memory Delay : allblocks_alteradspbuilder2/Memory Delay  BusType=Unsigned Integer  bwl=8  bwr=0  pipeline=640  pipeline_display=640  ram_type=AUTO  use_ena=on  use_sclr=off  allowFloatingPointOverride=on  logOutputs=off  logFile=C:\Users\ASUS\Desktop\sift_fpga_final\Octave_1\tb_octave1\octave1_hist%5Fbin_Line%5Fbuffer%5F5x5_Memory+Delay.fixedpointlog
  Memory Delay1 : allblocks_alteradspbuilder2/Memory Delay  BusType=Unsigned Integer  bwl=8  bwr=0  pipeline=640  pipeline_display=640  ram_type=AUTO  use_ena=on  use_sclr=off  allowFloatingPointOverride=on  logOutputs=off  logFile=C:\Users\ASUS\Desktop\sift_fpga_final\Octave_1\tb_octave1\octave1_hist%5Fbin_Line%5Fbuffer%5F5x5_Memory+Delay1.fixedpointlog
  Memory Delay2 : allblocks_alteradspbuilder2/Memory Delay  BusType=Unsigned Integer  bwl=8  bwr=0  pipeline=640  pipeline_display=640  ram_type=AUTO  use_ena=on  use_sclr=off  allowFloatingPointOverride=on  logOutputs=off  logFile=C:\Users\ASUS\Desktop\sift_fpga_final\Octave_1\tb_octave1\octave1_hist%5Fbin_Line%5Fbuffer%5F5x5_Memory+Delay2.fixedpointlog
  Memory Delay3 : allblocks_alteradspbuilder2/Memory Delay  BusType=Unsigned Integer  bwl=8  bwr=0  pipeline=640  pipeline_display=640  ram_type=AUTO  use_ena=on  use_sclr=off  allowFloatingPointOverride=on  logOutputs=off  logFile=C:\Users\ASUS\Desktop\sift_fpga_final\Octave_1\tb_octave1\octave1_hist%5Fbin_Line%5Fbuffer%5F5x5_Memory+Delay3.fixedpointlog
  Out00 : Outport
  Out01 : Outport  Port=2
  Out02 : Outport  Port=3
  Out03 : Outport  Port=4
  Out04 : Outport  Port=5
  Out10 : Outport  Port=6
  Out11 : Outport  Port=7
  Out12 : Outport  Port=8
  Out13 : Outport  Port=9
  Out14 : Outport  Port=10
  Out20 : Outport  Port=11
  Out21 : Outport  Port=12
  Out22 : Outport  Port=13
  Out23 : Outport  Port=14
  Out24 : Outport  Port=15
  Out30 : Outport  Port=16
  Out31 : Outport  Port=17
  Out32 : Outport  Port=18
  Out33 : Outport  Port=19
  Out34 : Outport  Port=20
  Out40 : Outport  Port=21
  Out41 : Outport  Port=22
  Out42 : Outport  Port=23
  Out43 : Outport  Port=24
  Out44 : Outport  Port=25
  wires:
  [clken] -> Delay11/2
  Delay11/1 -> [data_23], Delay12/1
  [clken] -> Delay12/2
  [clken] -> Delay10/2
  Delay8/1 -> Memory Delay1/1, [data_14]
  [clken] -> Memory Delay1/2
  Delay9/1 -> [data_21], Delay10/1
  Memory Delay1/1 -> [data_20], Delay9/1
  Delay10/1 -> [data_22], Delay11/1
  [clken] -> Delay9/2
  [clken] -> Delay4/2
  [data_03] -> Out03/1
  [data_04] -> Out04/1
  [data_02] -> Out02/1
  Delay/1 -> [data_00], Delay1/1
  [data_32] -> Out32/1
  [data_44] -> Out44/1
  [data_31] -> Out31/1
  [data_40] -> Out40/1
  [data_34] -> Out34/1
  [data_30] -> Out30/1
  [data_33] -> Out33/1
  [data_43] -> Out43/1
  [data_42] -> Out42/1
  [data_41] -> Out41/1
  [clken] -> Delay1/2
  [clken] -> Delay/2
  [data_in] -> Delay/1
  [clken] -> Delay2/2
  Delay2/1 -> [data_02], Delay3/1
  Delay1/1 -> [data_01], Delay2/1
  [clken] -> Delay3/2
  [data_01] -> Out01/1
  clken/1 -> [clken]
  [data_00] -> Out00/1
  [data_21] -> Out21/1
  [data_20] -> Out20/1
  [data_23] -> Out23/1
  [data_22] -> Out22/1
  [data_24] -> Out24/1
  dataIn/1 -> [data_in]
  [data_10] -> Out10/1
  [data_11] -> Out11/1
  [data_12] -> Out12/1
  [data_13] -> Out13/1
  [data_14] -> Out14/1
  Delay4/1 -> Memory Delay/1, [data_04]
  [clken] -> Memory Delay/2
  Delay12/1 -> [data_24], Memory Delay2/1
  [clken] -> Memory Delay2/2
  Memory Delay2/1 -> [data_30], Delay16/1
  [clken] -> Delay16/2
  [clken] -> Delay14/2
  [clken] -> Delay15/2
  [clken] -> Memory Delay3/2
  Delay17/1 -> [data_32], Delay18/1
  Delay18/1 -> [data_33], Delay19/1
  Memory Delay3/1 -> [data_40], Delay20/1
  [clken] -> Delay20/2
  [clken] -> Delay19/2
  Delay13/1 -> [data_42], Delay14/1
  Delay19/1 -> Memory Delay3/1, [data_34]
  Delay14/1 -> [data_43], Delay15/1
  Delay15/1 -> [data_44]
  [clken] -> Delay17/2
  [clken] -> Delay18/2
  [clken] -> Delay13/2
  Delay16/1 -> [data_31], Delay17/1
  Delay20/1 -> [data_41], Delay13/1
  Memory Delay/1 -> [data_10], Delay5/1
  [clken] -> Delay7/2
  [clken] -> Delay6/2
  Delay5/1 -> [data_11], Delay6/1
  [clken] -> Delay8/2
  [clken] -> Delay5/2
  Delay7/1 -> [data_13], Delay8/1
  Delay6/1 -> [data_12], Delay7/1
  Delay3/1 -> [data_03], Delay4/1
